simulink model "MRA_2013b"  (Simulink 8.2)
settings: Solver=ode45  SolverMode=SingleTasking  StartTime=0.0  StopTime=" tsim"  MaxStep=0.01  RelTol=1e-3
values from neighbouring files (symbols this model uses):
  c = 10    [SistemaMasaResorteAmortiguador.m]
  F = 1    [SistemaMasaResorteAmortiguador.m]
  k = 20    [SistemaMasaResorteAmortiguador.m]
  m = 2    [SistemaMasaResorteAmortiguador.m]
settings Model: Creator=Sergio  LastModifiedBy=Sergio  CovMetricSettings=dwe  CovHtmlReporting=off  covSaveCumulativeToWorkspaceVar=off  CovSaveSingleToWorkspaceVar=off  CovExternalEMLEnable=on
settings DataIOCC: LimitDataPoints=off  SaveFormat=StructureWithTime  SignalLoggingSaveFormat=Dataset
settings OptimizationCC: ExpressionDepthLimit=128
settings DebuggingCC: UnderspecifiedInitializationDetection=Simplified  MergeDetectMultiDrivingBlocksExec=error  SolverPrmCheckMsg=none  FcnCallInpInsideContextMsg=EnableAllAsError  FrameProcessingCompatibilityMsg=error  StateNameClashWarn=none  SFUnexpectedBacktrackingDiag=error  SFNoUnconditionalDefaultTransitionDiag=error
settings HardwareCC: ProdBitPerPointer=64  ProdLargestAtomicFloat=Float  ProdIntDivRoundTo=Zero  ProdEndianess=LittleEndian  ProdHWDeviceType=Specified
settings ModelReferenceCC: PropagateSignalLabelsOutOfModel=on
settings GRTTargetCC: CodeReplacementLibrary=C99 (ISO)  GeneratePreprocessorConditionals=Use local settings  CombineOutputUpdateFcns=on  GRTInterface=off

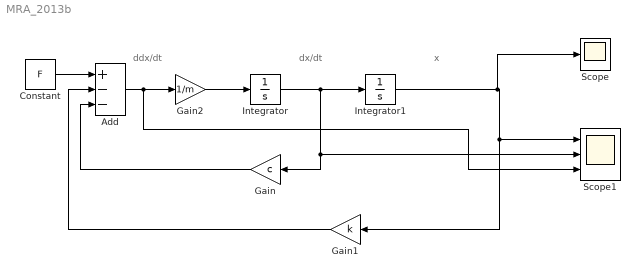
== system MRA_2013b ==
  note: ddx/dt
  note: dx/dt
  note: x
  Add : Sum  Inputs=+--
  Constant : Constant  Value=F
  Gain : Gain  Gain=c
  Gain1 : Gain  Gain=k
  Gain2 : Gain  Gain=1/m
  Integrator : Integrator
  Integrator1 : Integrator
  Scope : Scope
      settings: TimeRange=auto  MaxDataPoints=5000  SaveToWorkspace=off  SaveName=ScopeData  YMin=-0.00636  YMax=0.05722  SampleTime=-1
  Scope1 : Scope  NumInputPorts=3
      settings: TimeRange=auto  MaxDataPoints=5000  SaveToWorkspace=off  YMin=-0.00636~-0.00976~-0.33017  YMax=0.05722~0.07611~1.1478  SampleTime=-1
  wires:
  Gain2/1 -> Integrator/1
  Integrator/1 -> Scope1/2, Gain/1, Integrator1/1
  Constant/1 -> Add/1
  Gain/1 -> Add/3
  Integrator1/1 -> Scope/1, Scope1/1, Gain1/1
  Gain1/1 -> Add/2
  Add/1 -> Scope1/3, Gain2/1
